simulink model "Prac_1"  (R2023a)
settings: Solver=VariableStepAuto  StartTime=0.0  StopTime=500  MaxStep=0.001  RelTol=1e-3
model workspace (MAT data in the model file):
  K = Simulink.Parameter
  K.DataType = 'auto'
  K.Complexity = 'real'
  K.Dimensions = [0 0]
undefined symbols (not defined in the file): a_val, b, K_val
libraries: simulink x1
settings Model: Creator=Kae Young  LastModifiedBy=Kae Young

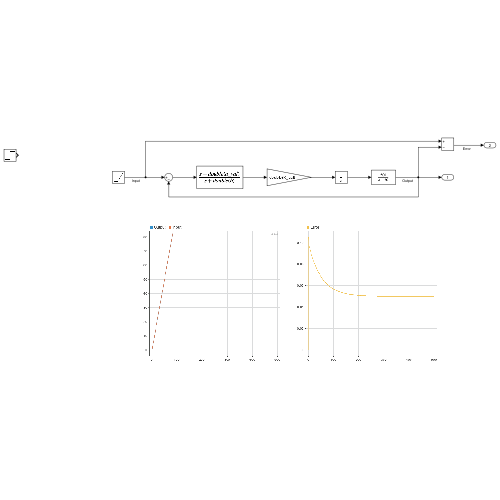
[thumbnail: Simulink's stored preview of the top-level diagram]
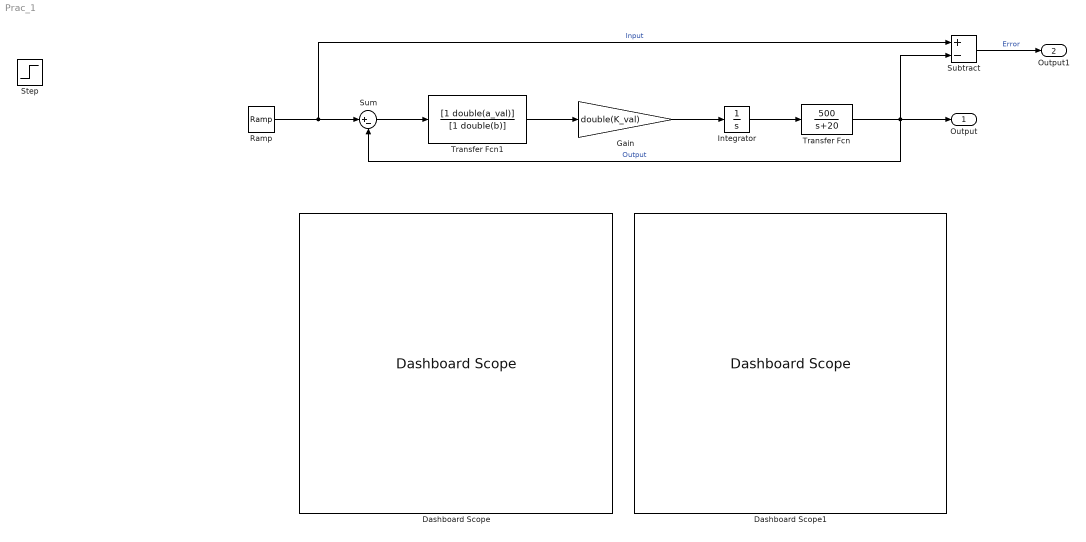
== system Prac_1 ==
  Dashboard Scope : DashboardScope
  Dashboard Scope1 : DashboardScope
  Gain : Gain  Gain=double(K_val)
  Integrator : Integrator
  Ramp : simulink/Sources/Ramp  slope=1  start=0  InitialOutput=0
  Step : Step  SampleTime=0
  Subtract : Sum  Inputs=+-
  Sum : Sum  Inputs=|+-
  Transfer Fcn : TransferFcn  Numerator=[500]  Denominator=[1 20]
  Transfer Fcn1 : TransferFcn  Numerator=[1 double(a_val)]  Denominator=[1 double(b)]
  Output : Outport
  Output1 : Outport  Port=2
  wires:
  Gain/1 -> Integrator/1
  Integrator/1 -> Transfer Fcn/1
  Transfer Fcn/1 -> Subtract/2, Sum/2, Output/1  "Output"
  Sum/1 -> Transfer Fcn1/1
  Transfer Fcn1/1 -> Gain/1
  Ramp/1 -> Subtract/1, Sum/1  "Input"
  Subtract/1 -> Output1/1  "Error"
